simulink model "Terminator1_Model"  (R2025a)
settings: Solver=VariableStepAuto  StartTime=0.0  StopTime=10.0  RelTol=1e-3
libraries: NSA_DEVS_SINKS x4, NSA_DEVS_SOURCES x2, TerminatorLib x1, NSA_DEVS_LOGISTICS x1
settings Model: Creator=david  LastModifiedBy=peter
settings RTWCC: GPUComputeCapability=3.5

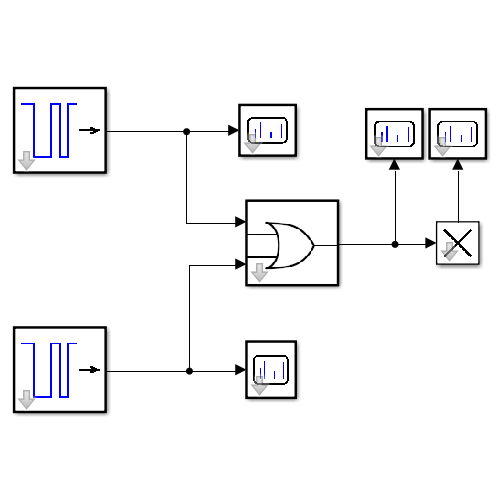
[thumbnail: Simulink's stored preview of the top-level diagram]
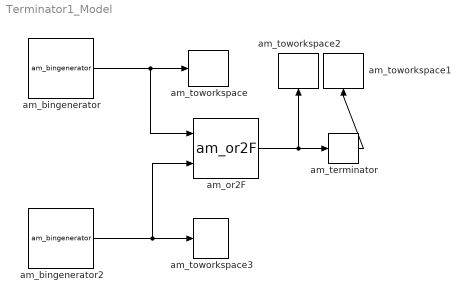
== system Terminator1_Model ==
  am_bingenerator : NSA_DEVS_SOURCES/am_bingenerator  z0=false  tVec=[1:8, 100]  tau=[0,1]  debug=0
      settings: SourceProductName=Sources
  am_bingenerator2 : NSA_DEVS_SOURCES/am_bingenerator  z0=false  tVec=[1:2:8, 100]  tau=[0,1]  debug=0
      settings: SourceProductName=Sources
  am_or2F : TerminatorLib/am_or2F  i0=false  tau_copy=[0,1]  debug_copy=0
  am_terminator : NSA_DEVS_LOGISTICS/am_terminator  countyEmptyInputs=true  tau_copy=[0,1]  debug_copy=0
      settings: SourceProductName=Logistics
  am_toworkspace : NSA_DEVS_SINKS/am_toworkspace  varname="\"gen1Out\""  t0=0  format="\"vector\""  tau=[0,5]  debug=0
      settings: SourceProductName=Sinks
  am_toworkspace1 : NSA_DEVS_SINKS/am_toworkspace  varname="\"nOut\""  t0=0  format="\"vector\""  tau=[0,5]  debug=0
      settings: SourceProductName=Sinks
  am_toworkspace2 : NSA_DEVS_SINKS/am_toworkspace  varname="\"orOut\""  t0=0  format="\"vector\""  tau=[0,5]  debug=0
      settings: SourceProductName=Sinks
  am_toworkspace3 : NSA_DEVS_SINKS/am_toworkspace  varname="\"gen2Out\""  t0=0  format="\"vector\""  tau=[0,5]  debug=0
      settings: SourceProductName=Sinks
  wires:
  am_bingenerator/1 -> am_or2F/1, am_toworkspace/1
  am_or2F/1 -> am_toworkspace2/1, am_terminator/1
  am_bingenerator2/1 -> am_or2F/2, am_toworkspace3/1
  am_terminator/1 -> am_toworkspace1/1
